simulink model "control_sim"  (R2021a)
settings: Solver=VariableStepAuto  StartTime=0.0  StopTime=10  RelTol=1e-3
undefined symbols (not defined in the file): A, B, C, D, K1, K2, K3
settings Model: Creator=1  LastModifiedBy=1

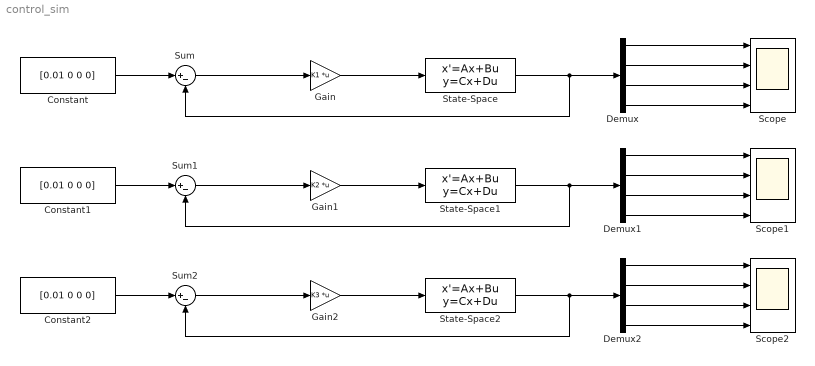
== system control_sim ==
  Constant : Constant  Value=[0.01 0 0 0]
  Constant1 : Constant  Value=[0.01 0 0 0]
  Constant2 : Constant  Value=[0.01 0 0 0]
  Demux : Demux
  Demux1 : Demux
  Demux2 : Demux
  Gain : Gain  Gain=K1  Multiplication=Matrix(K*u)
  Gain1 : Gain  Gain=K2  Multiplication=Matrix(K*u)
  Gain2 : Gain  Gain=K3  Multiplication=Matrix(K*u)
  Scope : Scope  NumInputPorts=4
  Scope1 : Scope  NumInputPorts=4
  Scope2 : Scope  NumInputPorts=4
  State-Space : StateSpace  A=A  B=B  C=C  D=D  InitialCondition=0
  State-Space1 : StateSpace  A=A  B=B  C=C  D=D  InitialCondition=0
  State-Space2 : StateSpace  A=A  B=B  C=C  D=D  InitialCondition=0
  Sum : Sum  Inputs=|+-
  Sum1 : Sum  Inputs=|+-
  Sum2 : Sum  Inputs=|+-
  wires:
  Gain/1 -> State-Space/1
  Sum/1 -> Gain/1
  Constant/1 -> Sum/1
  State-Space/1 -> Sum/2, Demux/1
  Demux/1 -> Scope/1
  Demux/2 -> Scope/2
  Demux/4 -> Scope/4
  Demux/3 -> Scope/3
  Demux1/2 -> Scope1/2
  Demux1/3 -> Scope1/3
  Constant1/1 -> Sum1/1
  Demux1/1 -> Scope1/1
  Gain1/1 -> State-Space1/1
  Sum1/1 -> Gain1/1
  State-Space1/1 -> Sum1/2, Demux1/1
  Demux1/4 -> Scope1/4
  Demux2/2 -> Scope2/2
  Demux2/3 -> Scope2/3
  Constant2/1 -> Sum2/1
  Demux2/1 -> Scope2/1
  Gain2/1 -> State-Space2/1
  Sum2/1 -> Gain2/1
  State-Space2/1 -> Sum2/2, Demux2/1
  Demux2/4 -> Scope2/4
